simulink model "Actuator"  (R2023a)
settings: Solver=FixedStepDiscrete  StartTime=0.0  StopTime=10.0  FixedStep=0.005  RelTol=1e-3
undefined symbols (not defined in the file): TPSPercentBkpt, TPSPercentTbl, Ts
settings Model: Creator=The MathWorks, Inc.  LastModifiedBy=omert
settings SolverCC: AlgebraicLoopSolver=TrustRegion
settings DataIOCC: SaveFormat=StructureWithTime
settings OptimizationCC: DefaultParameterBehavior=Inlined  EnhancedBackFolding=on  PassReuseOutputArgsAs=Individual arguments  ZeroExternalMemoryAtStartup=off  ZeroInternalMemoryAtStartup=off  OptimizeBlockOrder=speed  DifferentSizesBufferReuse=on  OptimizationCustomize=off  EfficientTunableParamExpr=on
settings DebuggingCC: ParameterTunabilityLossMsg=error  UnconnectedInputMsg=warning  UnconnectedOutputMsg=warning  UnconnectedLineMsg=warning
settings ModelReferenceCC: EnableRefExpFcnMdlSchedulingChecks=on
settings SFSimCC: MATLABDynamicMemAlloc=off
settings RTWCC: Description=Embedded Coder  SystemTargetFile=ert.tlc  GenCodeOnly=on  TemplateMakefile=ert_default_tmf  DLArmComputeVersion=19.05
settings CodeAppCC: ForceParamTrailComments=on  IgnoreCustomStorageClasses=off  MaxIdLength=255  OperatorAnnotations=on  SimulinkDataObjDesc=on  SFDataObjDesc=on  InsertBlockDesc=on
settings ERTTargetCC: TargetLangStandard=C99 (ISO)  GenerateSampleERTMain=on  InlinedParameterPlacement=NonHierarchical  ERTCustomFileTemplate=example_file_process.tlc

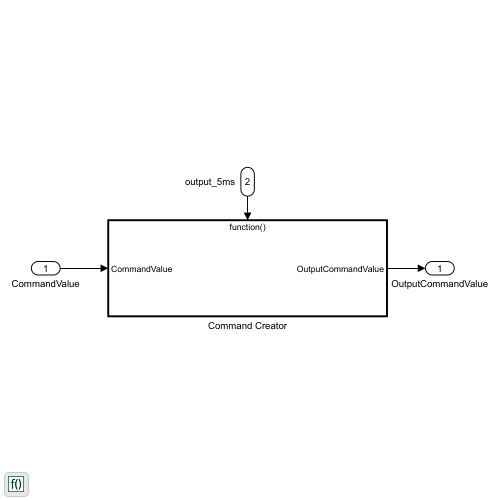
[thumbnail: Simulink's stored preview of the top-level diagram]
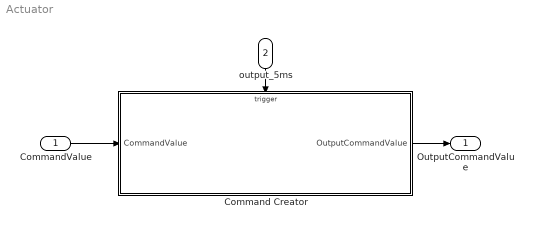
== system Actuator ==
  CommandValue : Inport  OutDataTypeStr=single  PortDimensions=1
  output_5ms : Inport  Port=2  OutputFunctionCall=on
  Command Creator : Subsystem  TreatAsAtomicUnit=on  SystemSampleTime=0.005
  OutputCommandValue : Outport  OutDataTypeStr=int16  PortDimensions=1
  wires:
  CommandValue/1 -> Command Creator/1(CommandValue)
  Command Creator/1(OutputCommandValue) -> OutputCommandValue/1
  output_5ms/1 -> Command Creator/Trigger

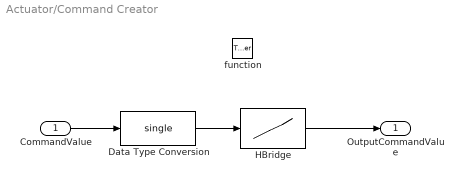
== system Actuator/Command Creator ==
  CommandValue : Inport
  function : TriggerPort  TriggerType=function-call  VariantControl=(inherit)  SampleTime=Ts  PortDimensions=1
  Data Type Conversion : DataTypeConversion  OutDataTypeStr=single  SaturateOnIntegerOverflow=off  RndMeth=Floor
  HBridge : Lookup_n-D  NumberOfTableDimensions=1  DataSpecification=Lookup table object  LookupTableObject=HBridge  BreakpointsForDimension1=TPSPercentBkpt  BreakpointsForDimension1DataTypeStr=single  IndexSearchMethod=Linear search  Table=TPSPercentTbl  TableDataTypeStr=single  InterpMethod=Nearest  InternalRulePriority=Speed  OutDataTypeStr=Inherit: Inherit from 'Table data'  RndMeth=Simplest
  OutputCommandValue : Outport
  wires:
  HBridge/1 -> OutputCommandValue/1
  Data Type Conversion/1 -> HBridge/1
  CommandValue/1 -> Data Type Conversion/1
